simulink model "RBCM_Model"  (R2024b)
settings: Solver=FixedStepAuto  StartTime=0.0  StopTime=10.0  RelTol=1e-3
PreLoadFcn:
  | % NXP_MBDT_S32K3 callback: DO NOT REMOVE
  | mbd_s32k3.common.nxp.model_callbacks.preLoadFcn();
PostLoadFcn:
  | % NXP_MBDT_S32K3 callback: DO NOT REMOVE
  | mbd_s32k3.common.nxp.model_callbacks.postLoadFcn();
InitFcn:
  | % NXP_MBDT_S32K3 callback: DO NOT REMOVE
  | mbd_s32k3.common.nxp.model_callbacks.initFcn();
undefined symbols (not defined in the file or in its folder): AccuFanPwr_hHsd3ch2, BspdPwr_lHsd1ch2, BuzzerPwr_lHsd3ch3, DevicePwr_12v_lHsd1ch1, DevicePwr_hHsd1ch2, DrsPwr_8v_lHsd3ch1, hHsd_Diagnose_AdcBuffer, ILPwr_hHsd1ch1, lHsd_Diagnose_AdcBuffer, LoggerPwr_lHsd1ch3, PumpFan1_hHsd4ch1, PumpFan2_hHsd4ch2, PumpPwr_hHsd3ch1, RGBLED0state, TaillightPwr_lHsd3ch4, TempSensorPwr_lHsd1ch4
libraries: mbd_s32k3_io_library x127, simulink x48, canmsglib x8, mbd_s32k3_communication_library x7, mbd_s32k3_isr_library x6, mbd_s32k3_cdd_library x3, mbd_s32k3_utility_library x1
(part 8 of 10)

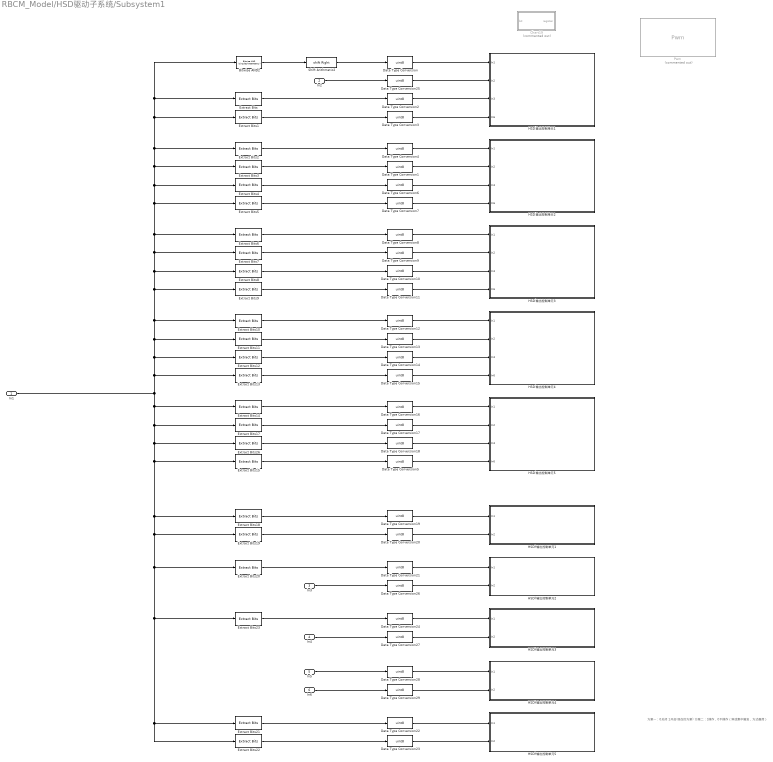
== system RBCM_Model/HSD驱动子系统/Subsystem1 ==
  note: 方案一：0关闭 1开启(现在的方案)
      | 方案二：1操作，0不操作（异或集中触发，方式最简）
  In1 : Inport  OutDataTypeStr=uint32
  In2 : Inport  Port=2  OutDataTypeStr=uint8
  In3 : Inport  Port=3  OutDataTypeStr=uint8
  In4 : Inport  Port=4  OutDataTypeStr=uint8
  In5 : Inport  Port=5  OutDataTypeStr=uint8
  In6 : Inport  Port=6  OutDataTypeStr=uint8
  Bitwise AND2 : simulink/Logic and Bit Operations/Bitwise Operator  logicop=AND  UseBitMask=on  BitMask=bin2dec('00000001')  BitMaskRealWorld=Stored Integer
      settings: LibrarySourceBlock=|
      | simulink/Quick Insert/Logic and Bit
      | Operations/Bitwise AND
  Chart19 : Stateflow chart  Commented=on  TreatAsAtomicUnit=on
  Data Type Conversion{,1..29} (30 alike) : DataTypeConversion  OutDataTypeStr=uint8  SaturateOnIntegerOverflow=off  RndMeth=Floor
  Extract Bits : simulink/Logic and Bit Operations/Extract Bits  bitsToExtract=Range of bits  numBits=8  bitIdxRange=[2 2]  outScalingMode=Preserve fixed-point scaling
  Extract Bits1 : simulink/Logic and Bit Operations/Extract Bits  bitsToExtract=Range of bits  numBits=8  bitIdxRange=[3 3]  outScalingMode=Preserve fixed-point scaling
  Extract Bits10 : simulink/Logic and Bit Operations/Extract Bits  bitsToExtract=Range of bits  numBits=8  bitIdxRange=[24 25]  outScalingMode=Preserve fixed-point scaling
  Extract Bits11 : simulink/Logic and Bit Operations/Extract Bits  bitsToExtract=Range of bits  numBits=8  bitIdxRange=[26 27]  outScalingMode=Preserve fixed-point scaling
  Extract Bits12 : simulink/Logic and Bit Operations/Extract Bits  bitsToExtract=Range of bits  numBits=8  bitIdxRange=[28 29]  outScalingMode=Preserve fixed-point scaling
  Extract Bits13 : simulink/Logic and Bit Operations/Extract Bits  bitsToExtract=Range of bits  numBits=8  bitIdxRange=[30 31]  outScalingMode=Preserve fixed-point scaling
  Extract Bits14 : simulink/Logic and Bit Operations/Extract Bits  bitsToExtract=Range of bits  numBits=8  bitIdxRange=[32 33]  outScalingMode=Preserve fixed-point scaling
  Extract Bits{15,18..23,26} (8 alike) : simulink/Logic and Bit Operations/Extract Bits  bitsToExtract=Range of bits  numBits=8  bitIdxRange=[36 37]  outScalingMode=Preserve fixed-point scaling
  Extract Bits17 : simulink/Logic and Bit Operations/Extract Bits  bitsToExtract=Range of bits  numBits=8  bitIdxRange=[34 35]  outScalingMode=Preserve fixed-point scaling
  Extract Bits2 : simulink/Logic and Bit Operations/Extract Bits  bitsToExtract=Range of bits  numBits=8  bitIdxRange=[4 4]  outScalingMode=Preserve fixed-point scaling
  Extract Bits3 : simulink/Logic and Bit Operations/Extract Bits  bitsToExtract=Range of bits  numBits=8  bitIdxRange=[5 5]  outScalingMode=Preserve fixed-point scaling
  Extract Bits4 : simulink/Logic and Bit Operations/Extract Bits  bitsToExtract=Range of bits  numBits=8  bitIdxRange=[6 6]  outScalingMode=Preserve fixed-point scaling
  Extract Bits5 : simulink/Logic and Bit Operations/Extract Bits  bitsToExtract=Range of bits  numBits=8  bitIdxRange=[7 7]  outScalingMode=Preserve fixed-point scaling
  Extract Bits6 : simulink/Logic and Bit Operations/Extract Bits  bitsToExtract=Range of bits  numBits=8  bitIdxRange=[16 17]  outScalingMode=Preserve fixed-point scaling
  Extract Bits7 : simulink/Logic and Bit Operations/Extract Bits  bitsToExtract=Range of bits  numBits=8  bitIdxRange=[18 19]  outScalingMode=Preserve fixed-point scaling
  Extract Bits8 : simulink/Logic and Bit Operations/Extract Bits  bitsToExtract=Range of bits  numBits=8  bitIdxRange=[20 21]  outScalingMode=Preserve fixed-point scaling
  Extract Bits9 : simulink/Logic and Bit Operations/Extract Bits  bitsToExtract=Range of bits  numBits=8  bitIdxRange=[22 23]  outScalingMode=Preserve fixed-point scaling
  HSDh输出控制单元1 : Subsystem
  HSDh输出控制单元2 : Subsystem
  HSDh输出控制单元3 : Subsystem
  HSDh输出控制单元4 : Subsystem
  HSDh输出控制单元5 : Subsystem
  HSDl输出控制单元1 : Subsystem
  HSDl输出控制单元2 : Subsystem
  HSDl输出控制单元3 : Subsystem
  HSDl输出控制单元4 : Subsystem
  HSDl输出控制单元5 : Subsystem
  Pwm : mbd_s32k3_io_library/Pwm  Commented=on  api_func=Pwm_SetDutyCycle  channel=PwmChannel_0  notification=PWM_RISING_EDGE  moduleId=PWM_EMIOS_INSTANCE_0  prescalerType=PWM_PRIMARY_PRESCALER  text=|
      | CommonPublishedInformation - CommonPublishedInformation Pwm 
      | CommonPublishedInformation/ArReleaseMajorVersion - 4 
      | CommonPublishedInformation/ArReleaseMinorVersion - 4 
      | CommonPublishedInformation/ArReleaseRevisionVersion - 0 
      | CommonPublishedInformation/ModuleId - 121 
      | CommonPublishedInformation/SwMajorVersion - 2 
      | CommonPublishedInformation/SwMinorVersion - 0 
      | CommonPublishedInformation/SwPatchVersion - 0 
      | CommonPublishedInformation/VendorId - 43 
      | IMPLEMENTATION-CONFIG-VARIANT - VARIANT-POST-BUILD 
      | POST_BUILD_VARIANT_USED - true 
      | PwmChannel - PwmChannel_0 PwmChannel_1 PwmChannel_2 PwmChannel_3 PwmChannel_4 PwmChannel_5 PwmChannel_6 PwmChannel_7 PwmChannel_8 
      | PwmChannel_0/Index - 0 
      | PwmChannel_0/PwmChannelId - 0 
      | PwmChannel_0/PwmDutycycleDefault - 2048 
      | PwmChannel_0/PwmHwChannel - /Pwm/Pwm/PwmChannelConfigSet/PwmEmios_0/PwmEmiosChannels_9 
      | PwmChannel_0/PwmIdleState - PWM_LOW 
      | PwmChannel_0/PwmMcuClockReferencePoint - /Mcu/Mcu/McuModuleConfiguration/McuClockSettingConfig_0/CORE_CLK 
      | PwmChannel_0/PwmNotification - PwmChannel_0_Callback 
      | PwmChannel_0/PwmPeriodDefault - 16000.0 
      | PwmChannel_0/PwmPeriodInTicks - true 
      | PwmChannel_0/PwmPolarity - PWM_HIGH 
      | PwmChannel_1/Index - 1 
      | PwmChannel_1/PwmChannelId - 1 
      | PwmChannel_1/PwmDutycycleDefault - 2048 
      | PwmChannel_1/PwmHwChannel - /Pwm/Pwm/PwmChannelConfigSet/PwmEmios_0/PwmEmiosChannels_17 
      | PwmChannel_1/PwmIdleState - PWM_LOW 
      | PwmChannel_1/PwmMcuClockReferencePoint - /Mcu/Mcu/McuModuleConfiguration/McuClockSettingConfig_0/CORE_CLK 
      | PwmChannel_1/PwmNotification - PwmChannel_1_Callback 
      | PwmChannel_1/PwmPeriodDefault - 16000.0 
      | PwmChannel_1/PwmPeriodInTicks - true 
      | PwmChannel_1/PwmPolarity - PWM_HIGH 
      | PwmChannel_2/Index - 2 
      | PwmChannel_2/PwmChannelId - 2 
      | PwmChannel_2/PwmDutycycleDefault - 0 
      | PwmChannel_2/PwmHwChannel - /Pwm/Pwm/PwmChannelConfigSet/PwmEmios_1/PwmEmiosChannels_19 
      | PwmChannel_2/PwmIdleState - PWM_LOW 
      | PwmChannel_2/PwmMcuClockReferencePoint - /Mcu/Mcu/McuModuleConfiguration/McuClockSettingConfig_0/CORE_CLK 
      | PwmChannel_2/PwmNotification - PwmChannel_2_Callback 
      | PwmChannel_2/PwmPeriodDefault - 16000.0 
      | PwmChannel_2/PwmPeriodInTicks - true 
      | PwmChannel_2/PwmPolarity - PWM_HIGH 
      | PwmChannel_3/Index - 3 
      | PwmChannel_3/PwmChannelId - 3 
      | PwmChannel_3/PwmDutycycleDefault - 0 
      | PwmChannel_3/PwmHwChannel - /Pwm/Pwm/PwmChannelConfigSet/PwmEmios_1/PwmEmiosChannels_20 
      | PwmChannel_3/PwmIdleState - PWM_LOW 
      | PwmChannel_3/PwmMcuClockReferencePoint - /Mcu/Mcu/McuModuleConfiguration/McuClockSettingConfig_0/CORE_CLK 
      | PwmChannel_3/PwmNotification - PwmChannel_3_Callback 
      | PwmChannel_3/PwmPeriodDefault - 16000.0 
      | PwmChannel_3/PwmPeriodInTicks - true 
      | PwmChannel_3/PwmPolarity - PWM_HIGH 
      | PwmChannel_4/Index - 4 
      | PwmChannel_4/PwmChannelId - 4 
      | PwmChannel_4/PwmDutycycleDefault - 0 
      | PwmChannel_4/PwmHwChannel - /Pwm/Pwm/PwmChannelConfigSet/PwmEmios_1/PwmEmiosChannels_0 
      | PwmChannel_4/PwmIdleState - PWM_LOW 
      | PwmChannel_4/PwmMcuClockReferencePoint - /Mcu/Mcu/McuModuleConfiguration/McuClockSettingConfig_0/CORE_CLK 
      | PwmChannel_4/PwmNotification - PwmChannel_4_Callback 
      | PwmChannel_4/PwmPeriodDefault - 16000.0 
      | PwmChannel_4/PwmPeriodInTicks - true 
      | PwmChannel_4/PwmPolarity - PWM_HIGH 
      | PwmChannel_5/Index - 5 
      | PwmChannel_5/PwmChannelId - 5 
      | PwmChannel_5/PwmDutycycleDefault - 0 
      | PwmChannel_5/PwmHwChannel - /Pwm/Pwm/PwmChannelConfigSet/PwmEmios_1/PwmEmiosChannels_1 
      | PwmChannel_5/PwmIdleState - PWM_LOW 
      | PwmChannel_5/PwmMcuClockReferencePoint - /Mcu/Mcu/McuModuleConfiguration/McuClockSettingConfig_0/CORE_CLK 
      | PwmChannel_5/PwmNotification - PwmChannel_5_Callback 
      | PwmChannel_5/PwmPeriodDefault - 16000.0 
      | PwmChannel_5/PwmPeriodInTicks - true 
      | PwmChannel_5/PwmPolarity - PWM_HIGH 
      | PwmChannel_6/Index - 6 
      | PwmChannel_6/PwmChannelId - 6 
      | PwmChannel_6/PwmDutycycleDefault - 0 
      | PwmChannel_6/PwmHwChannel - /Pwm/Pwm/PwmChannelConfigSet/PwmEmios_1/PwmEmiosChannels_21 
      | PwmChannel_6/PwmIdleState - PWM_LOW 
      | PwmChannel_6/PwmMcuClockReferencePoint - /Mcu/Mcu/McuModuleConfiguration/McuClockSettingConfig_0/CORE_CLK 
      | PwmChannel_6/PwmNotification - PwmChannel_6_Callback 
      | PwmChannel_6/PwmPeriodDefault - 16000.0 
      | PwmChannel_6/PwmPeriodInTicks - true 
      | PwmChannel_6/PwmPolarity - PWM_HIGH 
      | PwmChannel_7/Index - 7 
      | PwmChannel_7/PwmChannelId - 7 
      | PwmChannel_7/PwmDutycycleDefault - 0 
      | PwmChannel_7/PwmHwChannel - /Pwm/Pwm/PwmChannelConfigSet/PwmEmios_1/PwmEmiosChannels_22 
      | PwmChannel_7/PwmIdleState - PWM_LOW 
      | PwmChannel_7/PwmMcuClockReferencePoint - /Mcu/Mcu/McuModuleConfiguration/McuClockSettingConfig_0/CORE_CLK 
      | PwmChannel_7/PwmNotification - PwmChannel_7_Callback 
      | PwmChannel_7/PwmPeriodDefault - 16000.0 
      | PwmChannel_7/PwmPeriodInTicks - true 
      | PwmChannel_7/PwmPolarity - PWM_HIGH 
      | PwmChannel_8/Index - 8 
      | PwmChannel_8/PwmChannelId - 8 
      | PwmChannel_8/PwmDutycycleDefault - 0 
      | PwmChannel_8/PwmHwChannel - /Pwm/Pwm/PwmChannelConfigSet/PwmEmios_2/PwmEmiosChannels_7 
      | PwmChannel_8/PwmIdleState - PWM_LOW 
      | PwmChannel_8/PwmMcuClockReferencePoint - /Mcu/Mcu/McuModuleConfiguration/McuClockSettingConfig_0/CORE_CLK 
      | PwmChannel_8/PwmNotification - PwmChannel_8_Callback 
      | PwmChannel_8/PwmPeriodDefault - 40000 
      | PwmChannel_8/PwmPeriodInTicks - true 
      | PwmChannel_8/PwmPolarity - PWM_HIGH 
      | PwmConfigurationOfOptApiServices - PwmConfigurationOfOptApiServices 
      | PwmConfigurationOfOptApiServices/PwmDeInitApi - true 
      | PwmConfigurationOfOptApiServices/PwmEmiosFastUpdateApi - true 
      | PwmConfigurationOfOptApiServices/PwmEnableMaskOutputs - false 
      | PwmConfigurationOfOptApiServices/PwmGetChannelStateApi - true 
      | PwmConfigurationOfOptApiServices/PwmGetOutputState - true 
      | PwmConfigurationOfOptApiServices/PwmSetChannelDeadTime - true 
      | PwmConfigurationOfOptApiServices/PwmSetChannelOutputApi - true 
      | PwmConfigurationOfOptApiServices/PwmSetCounterBusApi - true 
      | PwmConfigurationOfOptApiServices/PwmSetDutyCycle - true 
      | PwmConfigurationOfOptApiServices/PwmSetDutyCycle_NoUpdate - false 
      | PwmConfigurationOfOptApiServices/PwmSetDutyPhaseShift - false 
      | PwmConfigurationOfOptApiServices/PwmSetOutputToIdle - true 
      | PwmConfigurationOfOptApiServices/PwmSetPeriodAndDuty - true 
      | PwmConfigurationOfOptApiServices/PwmSetPeriodAndDuty_NoUpdate - false 
      | PwmConfigurationOfOptApiServices/PwmSetTriggerDelayApi - true 
      | PwmConfigurationOfOptApiServices/PwmVersionInfoApi - true 
      | PwmEmios - PwmEmios_0 PwmEmios_1 PwmEmios_2 
      | PwmEmios_0/Index - 0 
      | PwmEmios_0/PwmEmiosChannels - PwmEmiosChannels_17 PwmEmiosChannels_9 
      | PwmEmios_0/PwmEmiosChannels_17/EmiosChCounterBus - EMIOS_PWM_IP_BUS_A 
      | PwmEmios_0/PwmEmiosChannels_17/EmiosChDeadtime - 0 
      | PwmEmios_0/PwmEmiosChannels_17/EmiosChFlagGeneration - Trailing_Edge 
      | PwmEmios_0/PwmEmiosChannels_17/EmiosChFreeze - false 
      | PwmEmios_0/PwmEmiosChannels_17/EmiosChId - CH_17 
      | PwmEmios_0/PwmEmiosChannels_17/EmiosChInterrupt - EMIOS_PWM_IP_INTERRUPT_REQUEST 
      | PwmEmios_0/PwmEmiosChannels_17/EmiosChMode - EMIOS_PWM_IP_MODE_OPWMB 
      | PwmEmios_0/PwmEmiosChannels_17/EmiosChOutputDisable - EMIOS_PWM_IP_OUTPUT_DISABLE_NONE 
      | PwmEmios_0/PwmEmiosChannels_17/EmiosChPhaseShift - 0 
      | PwmEmios_0/PwmEmiosChannels_17/EmiosChPrescaler - EMIOS_PWM_IP_CLOCK_DIV_2 
      | PwmEmios_0/PwmEmiosChannels_17/EmiosChPrescalerAlternate - EMIOS_PWM_IP_CLOCK_DIV_1 
      | PwmEmios_0/PwmEmiosChannels_17/EmiosChPrescalerSource - EMIOS_PWM_IP_PS_SRC_MODULE_CLOCK 
      | PwmEmios_0/PwmEmiosChannels_17/EmiosChTrigger - 0 
      | PwmEmios_0/PwmEmiosChannels_17/Index - 1 
      | PwmEmios_0/PwmEmiosChannels_17/PwmEmiosBusRef - /Mcl/Mcl/MclConfig/EmiosCommon_0/EmiosMclMasterBus_0 
      | PwmEmios_0/PwmEmiosChannels_9/EmiosChCounterBus - EMIOS_PWM_IP_BUS_A 
      | PwmEmios_0/PwmEmiosChannels_9/EmiosChDeadtime - 0 
      | PwmEmios_0/PwmEmiosChannels_9/EmiosChFlagGeneration - Trailing_Edge 
      | PwmEmios_0/PwmEmiosChannels_9/EmiosChFreeze - false 
      | PwmEmios_0/PwmEmiosChannels_9/EmiosChId - CH_9 
      | PwmEmios_0/PwmEmiosChannels_9/EmiosChInterrupt - EMIOS_PWM_IP_INTERRUPT_REQUEST 
      | PwmEmios_0/PwmEmiosChannels_9/EmiosChMode - EMIOS_PWM_IP_MODE_OPWMB 
      | PwmEmios_0/PwmEmiosChannels_9/EmiosChOutputDisable - EMIOS_PWM_IP_OUTPUT_DISABLE_NONE 
      | PwmEmios_0/PwmEmiosChannels_9/EmiosChPhaseShift - 0 
      | PwmEmios_0/PwmEmiosChannels_9/EmiosChPrescaler - EMIOS_PWM_IP_CLOCK_DIV_1 
      | PwmEmios_0/PwmEmiosChannels_9/EmiosChPrescalerAlternate - EMIOS_PWM_IP_CLOCK_DIV_1 
      | PwmEmios_0/PwmEmiosChannels_9/EmiosChPrescalerSource - EMIOS_PWM_IP_PS_SRC_MODULE_CLOCK 
      | PwmEmios_0/PwmEmiosChannels_9/EmiosChTrigger - 0 
      | PwmEmios_0/PwmEmiosChannels_9/Index - 0 
      | PwmEmios_0/PwmEmiosChannels_9/PwmEmiosBusRef - /Mcl/Mcl/MclConfig/EmiosCommon_0/EmiosMclMasterBus_0 
      | PwmEmios_0/PwmHwInstance - Emios_0 
      | PwmEmios_1/Index - 1 
      | PwmEmios_1/PwmEmiosChannels - PwmEmiosChannels_0 PwmEmiosChannels_1 PwmEmiosChannels_19 PwmEmiosChannels_20 PwmEmiosChannels_21 PwmEmiosChannels_22 
      | PwmEmios_1/PwmEmiosChannels_0/EmiosChCounterBus - EMIOS_PWM_IP_BUS_A 
      | PwmEmios_1/PwmEmiosChannels_0/EmiosChDeadtime - 0 
      | PwmEmios_1/PwmEmiosChannels_0/EmiosChFlagGeneration - Trailing_Edge 
      | PwmEmios_1/PwmEmiosChannels_0/EmiosChFreeze - false 
      | PwmEmios_1/PwmEmiosChannels_0/EmiosChId - CH_0 
      | PwmEmios_1/PwmEmiosChannels_0/EmiosChInterrupt - EMIOS_PWM_IP_INTERRUPT_REQUEST 
      | PwmEmios_1/PwmEmiosChannels_0/EmiosChMode - EMIOS_PWM_IP_MODE_OPWMB 
      | PwmEmios_1/PwmEmiosChannels_0/EmiosChOutputDisable - EMIOS_PWM_IP_OUTPUT_DISABLE_NONE 
      | PwmEmios_1/PwmEmiosChannels_0/EmiosChPhaseShift - 0 
      | PwmEmios_1/PwmEmiosChannels_0/EmiosChPrescaler - EMIOS_PWM_IP_CLOCK_DIV_1 
      | PwmEmios_1/PwmEmiosChannels_0/EmiosChPrescalerAlternate - EMIOS_PWM_IP_CLOCK_DIV_1 
      | PwmEmios_1/PwmEmiosChannels_0/EmiosChPrescalerSource - EMIOS_PWM_IP_PS_SRC_MODULE_CLOCK 
      | PwmEmios_1/PwmEmiosChannels_0/EmiosChTrigger - 0 
      | PwmEmios_1/PwmEmiosChannels_0/Index - 2 
      | PwmEmios_1/PwmEmiosChannels_0/PwmEmiosBusRef - /Mcl/Mcl/MclConfig/EmiosCommon_1/EmiosMclMasterBus_0 
      | PwmEmios_1/PwmEmiosChannels_1/EmiosChCounterBus - EMIOS_PWM_IP_BUS_A 
      | PwmEmios_1/PwmEmiosChannels_1/EmiosChDeadtime - 0 
      | PwmEmios_1/PwmEmiosChannels_1/EmiosChFlagGeneration - Trailing_Edge 
      | PwmEmios_1/PwmEmiosChannels_1/EmiosChFreeze - false 
      | PwmEmios_1/PwmEmiosChannels_1/EmiosChId - CH_1 
      | PwmEmios_1/PwmEmiosChannels_1/EmiosChInterrupt - EMIOS_PWM_IP_INTERRUPT_REQUEST 
      | PwmEmios_1/PwmEmiosChannels_1/EmiosChMode - EMIOS_PWM_IP_MODE_OPWMB 
      | PwmEmios_1/PwmEmiosChannels_1/EmiosChOutputDisable - EMIOS_PWM_IP_OUTPUT_DISABLE_NONE 
      | PwmEmios_1/PwmEmiosChannels_1/EmiosChPhaseShift - 0 
      | PwmEmios_1/PwmEmiosChannels_1/EmiosChPrescaler - EMIOS_PWM_IP_CLOCK_DIV_1 
      | PwmEmios_1/PwmEmiosChannels_1/EmiosChPrescalerAlternate - EMIOS_PWM_IP_CLOCK_DIV_1 
      | PwmEmios_1/PwmEmiosChannels_1/EmiosChPrescalerSource - EMIOS_PWM_IP_PS_SRC_MODULE_CLOCK 
      | PwmEmios_1/PwmEmiosChannels_1/EmiosChTrigger - 0 
      | PwmEmios_1/PwmEmiosChannels_1/Index - 3 
      | PwmEmios_1/PwmEmiosChannels_1/PwmEmiosBusRef - /Mcl/Mcl/MclConfig/EmiosCommon_1/EmiosMclMasterBus_0 
      | PwmEmios_1/PwmEmiosChannels_19/EmiosChCounterBus - EMIOS_PWM_IP_BUS_A 
      | PwmEmios_1/PwmEmiosChannels_19/EmiosChDeadtime - 0 
      | PwmEmios_1/PwmEmiosChannels_19/EmiosChFlagGeneration - Trailing_Edge 
      | PwmEmios_1/PwmEmiosChannels_19/EmiosChFreeze - false 
      | PwmEmios_1/PwmEmiosChannels_19/EmiosChId - CH_19 
      | PwmEmios_1/PwmEmiosChannels_19/EmiosChInterrupt - EMIOS_PWM_IP_INTERRUPT_REQUEST 
      | PwmEmios_1/PwmEmiosChannels_19/EmiosChMode - EMIOS_PWM_IP_MODE_OPWMB 
      | PwmEmios_1/PwmEmiosChannels_19/EmiosChOutputDisable - EMIOS_PWM_IP_OUTPUT_DISABLE_NONE 
      | PwmEmios_1/PwmEmiosChannels_19/EmiosChPhaseShift - 0 
      | PwmEmios_1/PwmEmiosChannels_19/EmiosChPrescaler - EMIOS_PWM_IP_CLOCK_DIV_1 
      | PwmEmios_1/PwmEmiosChannels_19/EmiosChPrescalerAlternate - EMIOS_PWM_IP_CLOCK_DIV_1 
      | PwmEmios_1/PwmEmiosChannels_19/EmiosChPrescalerSource - EMIOS_PWM_IP_PS_SRC_MODULE_CLOCK 
      | PwmEmios_1/PwmEmiosChannels_19/EmiosChTrigger - 0 
      | PwmEmios_1/PwmEmiosChannels_19/Index - 0 
      | PwmEmios_1/PwmEmiosChannels_19/PwmEmiosBusRef - /Mcl/Mcl/MclConfig/EmiosCommon_1/EmiosMclMasterBus_0 
      | PwmEmios_1/PwmEmiosChannels_20/EmiosChCounterBus - EMIOS_PWM_IP_BUS_A 
      | PwmEmios_1/PwmEmiosChannels_20/EmiosChDeadtime - 0 
      | PwmEmios_1/PwmEmiosChannels_20/EmiosChFlagGeneration - Trailing_Edge 
      | PwmEmios_1/PwmEmiosChannels_20/EmiosChFreeze - false 
      | PwmEmios_1/PwmEmiosChannels_20/EmiosChId - CH_20 
      | PwmEmios_1/PwmEmiosChannels_20/EmiosChInterrupt - EMIOS_PWM_IP_INTERRUPT_REQUEST 
      | PwmEmios_1/PwmEmiosChannels_20/EmiosChMode - EMIOS_PWM_IP_MODE_OPWMB 
      | PwmEmios_1/PwmEmiosChannels_20/EmiosChOutputDisable - EMIOS_PWM_IP_OUTPUT_DISABLE_NONE 
      | PwmEmios_1/PwmEmiosChannels_20/EmiosChPhaseShift - 0 
      | PwmEmios_1/PwmEmiosChannels_20/EmiosChPrescaler - EMIOS_PWM_IP_CLOCK_DIV_1 
      | PwmEmios_1/PwmEmiosChannels_20/EmiosChPrescalerAlternate - EMIOS_PWM_IP_CLOCK_DIV_1 
      | PwmEmios_1/PwmEmiosChannels_20/EmiosChPrescalerSource - EMIOS_PWM_IP_PS_SRC_MODULE_CLOCK 
      | PwmEmios_1/PwmEmiosChannels_20/EmiosChTrigger - 0 
      | PwmEmios_1/PwmEmiosChannels_20/Index - 1 
      | PwmEmios_1/PwmEmiosChannels_20/PwmEmiosBusRef - /Mcl/Mcl/MclConfig/EmiosCommon_1/EmiosMclMasterBus_0 
      | PwmEmios_1/PwmEmiosChannels_21/EmiosChCounterBus - EMIOS_PWM_IP_BUS_A 
      | PwmEmios_1/PwmEmiosChannels_21/EmiosChDeadtime - 0 
      | PwmEmios_1/PwmEmiosChannels_21/EmiosChFlagGeneration - Trailing_Edge 
      | PwmEmios_1/PwmEmiosChannels_21/EmiosChFreeze - false 
      | PwmEmios_1/PwmEmiosChannels_21/EmiosChId - CH_21 
      | PwmEmios_1/PwmEmiosChannels_21/EmiosChInterrupt - EMIOS_PWM_IP_INTERRUPT_REQUEST 
      | PwmEmios_1/PwmEmiosChannels_21/EmiosChMode - EMIOS_PWM_IP_MODE_OPWMB 
      | PwmEmios_1/PwmEmiosChannels_21/EmiosChOutputDisable - EMIOS_PWM_IP_OUTPUT_DISABLE_NONE 
      | PwmEmios_1/PwmEmiosChannels_21/EmiosChPhaseShift - 0 
      | PwmEmios_1/PwmEmiosChannels_21/EmiosChPrescaler - EMIOS_PWM_IP_CLOCK_DIV_1 
      | PwmEmios_1/PwmEmiosChannels_21/EmiosChPrescalerAlternate - EMIOS_PWM_IP_CLOCK_DIV_1 
      | PwmEmios_1/PwmEmiosChannels_21/EmiosChPrescalerSource - EMIOS_PWM_IP_PS_SRC_MODULE_CLOCK 
      | PwmEmios_1/PwmEmiosChannels_21/EmiosChTrigger - 0 
      | PwmEmios_1/PwmEmiosChannels_21/Index - 4 
      | PwmEmios_1/PwmEmiosChannels_21/PwmEmiosBusRef - /Mcl/Mcl/MclConfig/EmiosCommon_1/EmiosMclMasterBus_0 
      | PwmEmios_1/PwmEmiosChannels_22/EmiosChCounterBus - EMIOS_PWM_IP_BUS_A 
      | PwmEmios_1/PwmEmiosChannels_22/EmiosChDeadtime - 0 
      | PwmEmios_1/PwmEmiosChannels_22/EmiosChFlagGeneration - Trailing_Edge 
      | PwmEmios_1/PwmEmiosChannels_22/EmiosChFreeze - false 
      | PwmEmios_1/PwmEmiosChannels_22/EmiosChId - CH_22 
      | PwmEmios_1/PwmEmiosChannels_22/EmiosChInterrupt - EMIOS_PWM_IP_INTERRUPT_REQUEST 
      | PwmEmios_1/PwmEmiosChannels_22/EmiosChMode - EMIOS_PWM_IP_MODE_OPWMB 
      | PwmEmios_1/PwmEmiosChannels_22/EmiosChOutputDisable - EMIOS_PWM_IP_OUTPUT_DISABLE_NONE 
      | PwmEmios_1/PwmEmiosChannels_22/EmiosChPhaseShift - 0 
      | PwmEmios_1/PwmEmiosChannels_22/EmiosChPrescaler - EMIOS_PWM_IP_CLOCK_DIV_1 
      | PwmEmios_1/PwmEmiosChannels_22/EmiosChPrescalerAlternate - EMIOS_PWM_IP_CLOCK_DIV_1 
      | PwmEmios_1/PwmEmiosChannels_22/EmiosChPrescalerSource - EMIOS_PWM_IP_PS_SRC_MODULE_CLOCK 
      | PwmEmios_1/PwmEmiosChannels_22/EmiosChTrigger - 0 
      | PwmEmios_1/PwmEmiosChannels_22/Index - 5 
      | PwmEmios_1/PwmEmiosChannels_22/PwmEmiosBusRef - /Mcl/Mcl/MclConfig/EmiosCommon_1/EmiosMclMasterBus_0 
      | PwmEmios_1/PwmHwInstance - Emios_1 
      | PwmEmios_2/Index - 2 
      | PwmEmios_2/PwmEmiosChannels - PwmEmiosChannels_7 
      | PwmEmios_2/PwmEmiosChannels_7/EmiosChCounterBus - EMIOS_PWM_IP_BUS_A 
      | PwmEmios_2/PwmEmiosChannels_7/EmiosChDeadtime - 0 
      | PwmEmios_2/PwmEmiosChannels_7/EmiosChFlagGeneration - Trailing_Edge 
      | PwmEmios_2/PwmEmiosChannels_7/EmiosChFreeze - false 
      | PwmEmios_2/PwmEmiosChannels_7/EmiosChId - CH_7 
      | PwmEmios_2/PwmEmiosChannels_7/EmiosChInterrupt - EMIOS_PWM_IP_INTERRUPT_REQUEST 
      | PwmEmios_2/PwmEmiosChannels_7/EmiosChMode - EMIOS_PWM_IP_MODE_OPWMB 
      | PwmEmios_2/PwmEmiosChannels_7/EmiosChOutputDisable - EMIOS_PWM_IP_OUTPUT_DISABLE_NONE 
      | PwmEmios_2/PwmEmiosChannels_7/EmiosChPhaseShift - 0 
      | PwmEmios_2/PwmEmiosChannels_7/EmiosChPrescaler - EMIOS_PWM_IP_CLOCK_DIV_2 
      | PwmEmios_2/PwmEmiosChannels_7/EmiosChPrescalerAlternate - EMIOS_PWM_IP_CLOCK_DIV_2 
      | PwmEmios_2/PwmEmiosChannels_7/EmiosChPrescalerSource - EMIOS_PWM_IP_PS_SRC_MODULE_CLOCK 
      | PwmEmios_2/PwmEmiosChannels_7/EmiosChTrigger - 0 
      | PwmEmios_2/PwmEmiosChannels_7/Index - 0 
      | PwmEmios_2/PwmEmiosChannels_7/PwmEmiosBusRef - /Mcl/Mcl/MclConfig/EmiosCommon_2/EmiosMclMasterBus_0 
      | PwmEmios_2/PwmHwInstance - Emios_2 
      | PwmEtpu - PwmChannelConfigSet 
      | PwmGeneral - PwmGeneral 
      | PwmGeneral/PwmDevErrorDetect - true 
      | PwmGeneral/PwmDutycycleUpdatedEndperiod - false 
      | PwmGeneral/PwmEnableDualClockMode - false 
      | PwmGeneral/PwmEnableUserModeSupport - false 
      | PwmGeneral/PwmIndex - 0 
      | PwmGeneral/PwmMultiChannelSync - false 
      | PwmGeneral/PwmMultipartitionEnabled - false 
      | PwmGeneral/PwmNotificationSupported - true 
      | PwmGeneral/PwmPeriodUpdatedEndperiod - true
      settings: SourceProductName=IO Blocks
  Shift Arithmetic2 : ArithShift  BitShiftDirection=Right
  wires:
  Extract Bits22/1 -> Data Type Conversion23/1
  Data Type Conversion8/1 -> HSDl输出控制单元3/1(In1)
  Data Type Conversion23/1 -> HSDh输出控制单元5/2(In2)
  In5/1 -> Data Type Conversion28/1
  Data Type Conversion10/1 -> HSDl输出控制单元3/3(In3)
  Data Type Conversion3/1 -> HSDl输出控制单元1/4(In6)
  Data Type Conversion4/1 -> HSDl输出控制单元2/1(In1)
  Extract Bits8/1 -> Data Type Conversion10/1
  Extract Bits20/1 -> Data Type Conversion21/1
  Extract Bits2/1 -> Data Type Conversion4/1
  Data Type Conversion14/1 -> HSDl输出控制单元4/3(In3)
  Data Type Conversion6/1 -> HSDl输出控制单元2/3(In3)
  Extract Bits11/1 -> Data Type Conversion13/1
  Data Type Conversion15/1 -> HSDl输出控制单元4/4(In6)
  Extract Bits7/1 -> Data Type Conversion9/1
  Data Type Conversion27/1 -> HSDh输出控制单元3/2(In2)
  Extract Bits15/1 -> Data Type Conversion5/1
  Data Type Conversion22/1 -> HSDh输出控制单元5/1(In1)
  Data Type Conversion16/1 -> HSDl输出控制单元5/1(In1)
  Extract Bits5/1 -> Data Type Conversion7/1
  In2/1 -> Data Type Conversion25/1
  Data Type Conversion18/1 -> HSDl输出控制单元5/3(In3)
  Extract Bits26/1 -> Data Type Conversion18/1
  Extract Bits3/1 -> Data Type Conversion1/1
  In6/1 -> Data Type Conversion29/1
  Data Type Conversion/1 -> HSDl输出控制单元1/1(In1)
  Data Type Conversion24/1 -> HSDh输出控制单元3/1(In1)
  Data Type Conversion1/1 -> HSDl输出控制单元2/2(In2)
  Bitwise AND2/1 -> Shift Arithmetic2/1
  Extract Bits9/1 -> Data Type Conversion11/1
  Data Type Conversion9/1 -> HSDl输出控制单元3/2(In2)
  Extract Bits14/1 -> Data Type Conversion16/1
  Data Type Conversion21/1 -> HSDh输出控制单元2/1(In1)
  Data Type Conversion17/1 -> HSDl输出控制单元5/2(In2)
  Data Type Conversion19/1 -> HSDh输出控制单元1/1(In1)
  Data Type Conversion26/1 -> HSDh输出控制单元2/2(In2)
  Extract Bits21/1 -> Data Type Conversion22/1
  Shift Arithmetic2/1 -> Data Type Conversion/1
  Data Type Conversion5/1 -> HSDl输出控制单元5/4(In6)
  Extract Bits13/1 -> Data Type Conversion15/1
  Data Type Conversion7/1 -> HSDl输出控制单元2/4(In6)
  Extract Bits18/1 -> Data Type Conversion19/1
  Data Type Conversion11/1 -> HSDl输出控制单元3/4(In6)
  Extract Bits1/1 -> Data Type Conversion3/1
  Extract Bits4/1 -> Data Type Conversion6/1
  In1/1 -> Extract Bits26/1, Extract Bits15/1, Extract Bits18/1, Extract Bits22/1, Extract Bits21/1, Extract Bits23/1, Extract Bits20/1, Extract Bits19/1, Extract Bits17/1, Extract Bits14/1, Extract Bits13/1, Extract Bits12/1, Extract Bits11/1, Extract Bits10/1, Extract Bits9/1, Extract Bits8/1, Extract Bits7/1, Extract Bits6/1, Extract Bits5/1, Extract Bits4/1, Extract Bits3/1, Extract Bits2/1, Extract Bits/1, Bitwise AND2/1, Extract Bits1/1
  Extract Bits17/1 -> Data Type Conversion17/1
  Data Type Conversion2/1 -> HSDl输出控制单元1/3(In3)
  Data Type Conversion25/1 -> HSDl输出控制单元1/2(In2)
  Data Type Conversion29/1 -> HSDh输出控制单元4/2(In2)
  Extract Bits19/1 -> Data Type Conversion20/1
  Extract Bits/1 -> Data Type Conversion2/1
  Extract Bits6/1 -> Data Type Conversion8/1
  Data Type Conversion28/1 -> HSDh输出控制单元4/1(In1)
  Extract Bits12/1 -> Data Type Conversion14/1
  Data Type Conversion12/1 -> HSDl输出控制单元4/1(In1)
  In4/1 -> Data Type Conversion27/1
  Extract Bits23/1 -> Data Type Conversion24/1
  Extract Bits10/1 -> Data Type Conversion12/1
  In3/1 -> Data Type Conversion26/1
  Data Type Conversion13/1 -> HSDl输出控制单元4/2(In2)
  Data Type Conversion20/1 -> HSDh输出控制单元1/2(In2)

== system RBCM_Model/Subsystem13/Subsystem ==
  Action Port : ActionPort  ActionPortLabel=else
  HsdDriveCommand Struct1 : MATLAB Function  TreatAsAtomicUnit=on
  y : Outport
  wires:
  HsdDriveCommand Struct1/1(HsdDriveCommands) -> y/1

== system RBCM_Model/Subsystem13/Subsystem13 ==
  In1 : Inport
  Action Port : ActionPort  ActionPortLabel=if(u1 > 0)
  Out1 : Outport
  wires:
  In1/1 -> Out1/1

== system RBCM_Model/Subsystem5/Subsystem ==
  Action Port : ActionPort  ActionPortLabel=else
  MATLAB Function : MATLAB Function  TreatAsAtomicUnit=on
  y : Outport
  wires:
  MATLAB Function/1(y) -> y/1

== system RBCM_Model/Subsystem5/Subsystem13 ==
  In1 : Inport
  Action Port : ActionPort  ActionPortLabel=if(u1 > 0)
  Out1 : Outport
  wires:
  In1/1 -> Out1/1

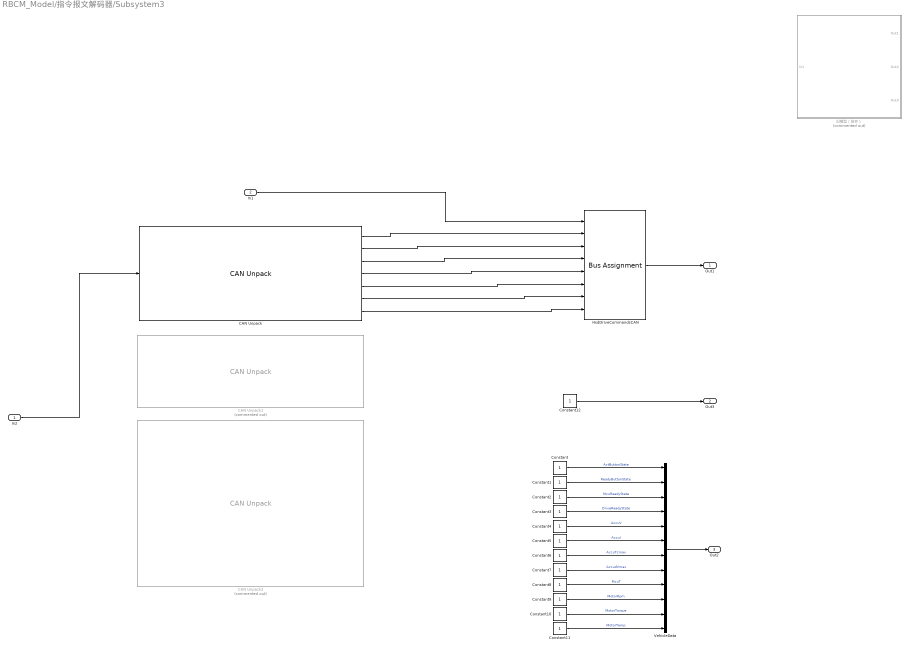
== system RBCM_Model/指令报文解码器/Subsystem3 ==
  In2 : Inport  OutDataTypeStr=Bus: Bus_CAN_RX_MESSAG
  In1 : Inport  Port=2
  CAN Unpack : canmsglib/CAN Unpack  CANdbFile=E:\Workspace\Myworkspace\RBCM_S32K344_AUTOSAR_MBD\Firmware\AUTOSAR_MBD\RBCM_ModelConfig\E10_dbc_240819_CAN.dbc  MsgList=PDB_ctr  MsgName=PDB_ctr  MsgIDType=Extended (29-bit identifier)  MsgIdentifier=514  MsgLength=8  SignalInfo={'Beep','2','2','LE','unsigned','Standard','0','1','0','0','2';'DRS','0','2','LE','unsigned','Standard','0','1','0','0','2';'FAN1','8','8','LE','unsigned','Standard','0','1','0','0','100';'FAN2','16','8','LE','unsigned','Standard','0','1','0','0','100';'FAN3','24','8','LE','unsigned','Standard','0','1','0','0','100';'Pump','40','8','LE','unsigned','Standard','0','1','0','0','100';'Taillight','32','8','LE','unsigned','Standard','0','1','0','0','100'}  IDPort=off  TimestampPort=off  ErrorPort=off  RemotePort=off  LengthPort=off  StatusPort=off  ApplyMinMax=off
      settings: LibrarySourceBlock=canlib/CAN Unpack  DataFormat=CANdb specified signals
  CAN Unpack1 : canmsglib/CAN Unpack  Commented=on  CANdbFile=E:\WUTE\整车CAN通信\E10_240721.dbc  MsgList=(none)  MsgName=MCU_Pwr  MsgIDType=Extended (29-bit identifier)  MsgIdentifier=218089455  MsgLength=8  SignalInfo={'MCU_HvAcCurrRms','48','16','LE','unsigned','Standard','0','0.1','-1600','-1600','1600';'MCU_HvCurr','32','16','LE','unsigned','Standard','0','0.1','-1600','-1600','1600';'MCU_HvVolt','16','16','LE','unsigned','Standard','0','0.1','0','0','1000';'MCU_McuTemp','0','8','LE','unsigned','Standard','0','1','-50','-50','205';'MCU_MotorTemp','8','8','LE','unsigned','Standard','0','1','-50','-50','205'}  IDPort=off  TimestampPort=off  ErrorPort=off  RemotePort=off  LengthPort=off  StatusPort=off  ApplyMinMax=off
      settings: LibrarySourceBlock=canlib/CAN Unpack  DataFormat=CANdb specified signals
  CAN Unpack2 : canmsglib/CAN Unpack  Commented=on  CANdbFile=E:\WUTE\整车CAN通信\E10_240721.dbc  MsgList=(none)  MsgName=MCU_Stat  MsgIDType=Extended (29-bit identifier)  MsgIdentifier=218089199  MsgLength=8  SignalInfo={'MCU_AlmLv','56','2','LE','unsigned','Standard','0','1','0','0','3';'MCU_IsBrakeMode','35','1','LE','unsigned','Standard','0','1','0','0','1';'MCU_IsFreeMode','32','1','LE','unsigned','Standard','0','1','0','0','1';'MCU_IsHvOvervoltage','44','1','LE','unsigned','Standard','0','1','0','0','1';'MCU_IsHvUndervoltage','46','1','LE','unsigned','Standard','0','1','0','0','1';'MCU_IsLvError','45','1','LE','unsigned','Standard','0','1','0','0','1';'MCU_IsMcuNOTActive','39','1','LE','unsigned','Standard','0','1','0','0','1';'MCU_IsMcuOvertemp','48','1','LE','unsigned','Standard','0','1','0','0','1';'MCU_IsMotorOvertemp','49','1','LE','unsigned','Standard','0','1','0','0','1';'MCU_IsOverCurr','43','1','LE','unsigned','Standard','0','1','0','0','1';'MCU_IsPreChg','41','1','LE','unsigned','Standard','0','1','0','0','255';'MCU_IsReady','40','1','LE','unsigned','Standard','0','1','0','0','1';'MCU_IsRevoloverError','42','1','LE','unsigned','Standard','0','1','0','0','1';'MCU_IsSelfcheckPass','55','1','LE','unsigned','Standard','0','1','0','0','1';'MCU_IsSpdMode','34','1','LE','unsigned','Standard','0','1','0','0','1';'MCU_IsTorqMode','33','1','LE','unsigned','Standard','0','1','0','0','1';'MCU_IsUnderPowerLim','47','1','LE','unsigned','Standard','0','1','0','0','1';'MCU_IsZeroLocMode','36','1','LE','unsigned','Standard','0','1','0','0','1';'MCU_SPD_RPT','0','16','LE','unsigned','Standard','0','0.5','-10000','-10000','10000';'MCU_TORQ_RPT','16','16','LE','unsigned','Standard','0','1','0','0','1000'}  IDPort=off  TimestampPort=off  ErrorPort=off  RemotePort=off  LengthPort=off  StatusPort=off  ApplyMinMax=off
      settings: LibrarySourceBlock=canlib/CAN Unpack  DataFormat=CANdb specified signals
  Constant{,1..3,12} (5 alike) : Constant  OutDataTypeStr=uint8
  Constant{4..11} (8 alike) : Constant  OutDataTypeStr=uint16
  HsdDriveCommandsCAN : BusAssignment  AssignedSignals=BuzzerPwr_lHsd3ch3,DrsPwr_8v_lHsd3ch1,AccuFanPwr_hHsd3ch2,PumpFan1_hHsd4ch1,PumpFan2_hHsd4ch2,PumpPwr_hHsd3ch1,TaillightPwr_lHsd3ch4
  VehicleData : BusCreator  Inputs=12  OutDataTypeStr=Bus: Bus_Vehicle_Data  NonVirtualBus=on
      settings: InheritFromInputs=off
  旧模型（放弃） : Subsystem  Commented=on
  Out1 : Outport
  Out3 : Outport  Port=2
  Out2 : Outport  Port=3
  wires:
  In2/1 -> CAN Unpack/1
  In1/1 -> HsdDriveCommandsCAN/1
  CAN Unpack/1 -> HsdDriveCommandsCAN/2
  CAN Unpack/2 -> HsdDriveCommandsCAN/3
  CAN Unpack/3 -> HsdDriveCommandsCAN/4
  CAN Unpack/4 -> HsdDriveCommandsCAN/5
  CAN Unpack/5 -> HsdDriveCommandsCAN/6
  CAN Unpack/6 -> HsdDriveCommandsCAN/7
  CAN Unpack/7 -> HsdDriveCommandsCAN/8
  HsdDriveCommandsCAN/1 -> Out1/1
  VehicleData/1 -> Out2/1
  Constant/1 -> VehicleData/1  "ActButtonState"
  Constant1/1 -> VehicleData/2  "ReadyButtonState"
  Constant2/1 -> VehicleData/3  "McuReadyState"
  Constant3/1 -> VehicleData/4  "DriveReadyState"
  Constant4/1 -> VehicleData/5  "AccuV"
  Constant5/1 -> VehicleData/6  "AccuI"
  Constant6/1 -> VehicleData/7  "AccuTcmax"
  Constant7/1 -> VehicleData/8  "AccudVmax"
  Constant8/1 -> VehicleData/9  "McuT"
  Constant9/1 -> VehicleData/10  "MotorRpm"
  Constant10/1 -> VehicleData/11  "MotorTorque"
  Constant11/1 -> VehicleData/12  "MotorTemp"
  Constant12/1 -> Out3/1

== system RBCM_Model/无线调试模式管理子系统/Subsystem ==
  Action Port : ActionPort  ActionPortLabel=if(u1 == 0)
  Constant : Constant  OutDataTypeStr=uint8
  Constant1 : Constant  OutDataTypeStr=uint8
  Dio : mbd_s32k3_io_library/Dio  api_func=Dio_WriteChannel  channel=ESP32S3_EN_RESET  channel_group=No channel groups configured  port=PTB_H  gpioSim=on  text=<binary blob, 15399 chars, not shown>
      settings: SourceProductName=IO Blocks
  Dio1 : mbd_s32k3_io_library/Dio  api_func=Dio_WriteChannel  channel=ESP32S3_EN_SET  channel_group=No channel groups configured  port=PTB_H  gpioSim=on  text=<binary blob, 15399 chars, not shown>
      settings: SourceProductName=IO Blocks
  wires:
  Constant/1 -> Dio/1
  Constant1/1 -> Dio1/1

== system RBCM_Model/无线调试模式管理子系统/Subsystem1 ==
  Action Port : ActionPort  ActionPortLabel=else
  Constant : Constant  Value=0  OutDataTypeStr=uint8
  Dio : mbd_s32k3_io_library/Dio  api_func=Dio_WriteChannel  channel=ESP32S3_EN_RESET  channel_group=No channel groups configured  port=PTB_H  gpioSim=on  text=<binary blob, 15399 chars, not shown>
      settings: SourceProductName=IO Blocks
  wires:
  Constant/1 -> Dio/1

== system RBCM_Model/HSD诊断分析子系统/旧模型/ADC采集与处理单元11 ==
  note: 计算设备工作电流
  note: 计算ADC输入实际电压
  note: 计算设备功耗
  function : TriggerPort  TriggerType=function-call  VariantControl=Variant
  ADC resolution : Constant  Value=0b111111111111  OutDataTypeStr=uint16
  Data Store Read : DataStoreRead  DataStoreName=hHsd_Diagnose_AdcBuffer  DataStoreElements=hHsd_Diagnose_AdcBuffer(1)  IndexOptions=Index vector (dialog)  Indices=1  OutputSizes=1
  Data Type Conversion : DataTypeConversion  OutDataTypeStr=single  SaturateOnIntegerOverflow=off  RndMeth=Floor
  Divide : Product  Inputs=*/  OutDataTypeStr=single
  Magnification : Gain  Gain=1450  OutDataTypeStr=uint8
  Product : Product  OutDataTypeStr=single
  Product1 : Product  OutDataTypeStr=single
  Product2 : Product  OutDataTypeStr=single
  Ris : Constant  Value=650  OutDataTypeStr=uint16
  Subtract : Sum  Inputs=+-
  Terminator7 : Terminator
  Vbat : Constant  Value=28  OutDataTypeStr=uint16
  Vref : Constant  Value=5  OutDataTypeStr=uint8
  compensate : Constant  Value=0.05  OutDataTypeStr=single
  u : Outport
  wires:
  Data Store Read/1 -> Data Type Conversion/1
  Data Type Conversion/1 -> Product/1
  Product2/1 -> Terminator7/1  "device power value"
  compensate/1 -> Subtract/2
  Product1/1 -> Divide/1  "Actual voltage"
  Vbat/1 -> Subtract/1
  Product/1 -> Product1/2
  Vref/1 -> Product1/1
  Subtract/1 -> Product2/2
  Divide/1 -> Magnification/1
  Ris/1 -> Divide/2
  ADC resolution/1 -> Product/2
  Magnification/1 -> u/1, Product2/1  "device current value"

== system RBCM_Model/HSD诊断分析子系统/旧模型/ADC采集与处理单元2 ==
  note: 计算ADC输入实际电压
  note: 计算设备工作电流*10
  note: 计算设备功耗
  function : TriggerPort  TriggerType=function-call  VariantControl=Variant
  ADC resolution : Constant  Value=0b111111111111  OutDataTypeStr=uint16
  Data Store Read : DataStoreRead  DataStoreName=lHsd_Diagnose_AdcBuffer  DataStoreElements=lHsd_Diagnose_AdcBuffer(2)  IndexOptions=Index vector (dialog)  Indices=1  OutputSizes=1
  Data Type Conversion : DataTypeConversion  OutDataTypeStr=single  SaturateOnIntegerOverflow=off  RndMeth=Floor
  Divide : Product  Inputs=*/  OutDataTypeStr=single
  Magnification : Gain  Gain=300  OutDataTypeStr=uint8
  Product : Product  OutDataTypeStr=single
  Product1 : Product  OutDataTypeStr=single
  Product2 : Product  OutDataTypeStr=single
  Ris : Constant  Value=650  OutDataTypeStr=uint16
  Subtract : Sum  Inputs=+-
  Terminator7 : Terminator
  Vbat : Constant  Value=28  OutDataTypeStr=uint16
  Vref : Constant  Value=5  OutDataTypeStr=uint8
  compensate : Constant  Value=0.05  OutDataTypeStr=single
  u1 : Outport  OutDataTypeStr=uint8
  wires:
  Data Type Conversion/1 -> Product/1
  Product2/1 -> Terminator7/1  "device power value"
  Subtract/1 -> Product2/2
  compensate/1 -> Subtract/2
  Vbat/1 -> Subtract/1
  ADC resolution/1 -> Product/2
  Product/1 -> Product1/2
  Vref/1 -> Product1/1
  Product1/1 -> Divide/1  "Actual voltage"
  Ris/1 -> Divide/2
  Divide/1 -> Magnification/1
  Magnification/1 -> Product2/1, u1/1  "device current value"
  Data Store Read/1 -> Data Type Conversion/1

== system RBCM_Model/HSD诊断分析子系统/旧模型/ADC采集与处理单元3 ==
  note: 计算设备功耗
  note: 计算设备工作电流*10
  note: 计算ADC输入实际电压
  function : TriggerPort  TriggerType=function-call  VariantControl=Variant
  ADC resolution : Constant  Value=0b111111111111  OutDataTypeStr=uint16
  Data Store Read : DataStoreRead  DataStoreName=lHsd_Diagnose_AdcBuffer  DataStoreElements=lHsd_Diagnose_AdcBuffer(3)  IndexOptions=Index vector (dialog)  Indices=1  OutputSizes=1
  Data Type Conversion : DataTypeConversion  OutDataTypeStr=single  SaturateOnIntegerOverflow=off  RndMeth=Floor
  Divide : Product  Inputs=*/  OutDataTypeStr=single
  Magnification : Gain  Gain=300  OutDataTypeStr=uint8
  Product : Product  OutDataTypeStr=single
  Product1 : Product  OutDataTypeStr=single
  Product2 : Product  OutDataTypeStr=single
  Ris : Constant  Value=650  OutDataTypeStr=uint16
  Subtract : Sum  Inputs=+-
  Terminator7 : Terminator
  Vbat : Constant  Value=28  OutDataTypeStr=uint16
  Vref : Constant  Value=5  OutDataTypeStr=uint8
  compensate : Constant  Value=0.05  OutDataTypeStr=single
  u1 : Outport  OutDataTypeStr=uint8
  wires:
  Magnification/1 -> u1/1, Product2/1  "device current value"
  Divide/1 -> Magnification/1
  Ris/1 -> Divide/2
  Product1/1 -> Divide/1  "Actual voltage"
  Vref/1 -> Product1/1
  Product/1 -> Product1/2
  ADC resolution/1 -> Product/2
  Data Store Read/1 -> Data Type Conversion/1
  Vbat/1 -> Subtract/1
  compensate/1 -> Subtract/2
  Subtract/1 -> Product2/2
  Product2/1 -> Terminator7/1  "device power value"
  Data Type Conversion/1 -> Product/1

== system RBCM_Model/HSD诊断分析子系统/旧模型/ADC采集与处理单元4 ==
  note: 计算ADC输入实际电压
  note: 计算设备工作电流*10
  note: 计算设备功耗
  function : TriggerPort  TriggerType=function-call  VariantControl=Variant
  ADC resolution : Constant  Value=0b111111111111  OutDataTypeStr=uint16
  Data Store Read : DataStoreRead  DataStoreName=lHsd_Diagnose_AdcBuffer  DataStoreElements=lHsd_Diagnose_AdcBuffer(4)  IndexOptions=Index vector (dialog)  Indices=1  OutputSizes=1
  Data Type Conversion : DataTypeConversion  OutDataTypeStr=single  SaturateOnIntegerOverflow=off  RndMeth=Floor
  Divide : Product  Inputs=*/  OutDataTypeStr=single
  Magnification : Gain  Gain=300  OutDataTypeStr=uint8
  Product : Product  OutDataTypeStr=single
  Product1 : Product  OutDataTypeStr=single
  Product2 : Product  OutDataTypeStr=single
  Ris : Constant  Value=650  OutDataTypeStr=uint16
  Subtract : Sum  Inputs=+-
  Terminator7 : Terminator
  Vbat : Constant  Value=28  OutDataTypeStr=uint16
  Vref : Constant  Value=5  OutDataTypeStr=uint8
  compensate : Constant  Value=0.05  OutDataTypeStr=single
  u1 : Outport  OutDataTypeStr=uint8
  wires:
  Data Type Conversion/1 -> Product/1
  Product2/1 -> Terminator7/1  "device power value"
  Subtract/1 -> Product2/2
  compensate/1 -> Subtract/2
  Vbat/1 -> Subtract/1
  Data Store Read/1 -> Data Type Conversion/1
  ADC resolution/1 -> Product/2
  Product/1 -> Product1/2
  Vref/1 -> Product1/1
  Product1/1 -> Divide/1  "Actual voltage"
  Ris/1 -> Divide/2
  Divide/1 -> Magnification/1
  Magnification/1 -> Product2/1, u1/1  "device current value"

== system RBCM_Model/HSD诊断分析子系统/旧模型/ADC采集与处理单元5 ==
  note: 计算设备功耗
  note: 计算设备工作电流*10
  note: 计算ADC输入实际电压
  function : TriggerPort  TriggerType=function-call  VariantControl=Variant
  ADC resolution : Constant  Value=0b111111111111  OutDataTypeStr=uint16
  Data Store Read : DataStoreRead  DataStoreName=lHsd_Diagnose_AdcBuffer  DataStoreElements=lHsd_Diagnose_AdcBuffer(5)  IndexOptions=Index vector (dialog)  Indices=1  OutputSizes=1
  Data Type Conversion : DataTypeConversion  OutDataTypeStr=single  SaturateOnIntegerOverflow=off  RndMeth=Floor
  Divide : Product  Inputs=*/  OutDataTypeStr=single
  Magnification : Gain  Gain=300  OutDataTypeStr=uint8
  Product : Product  OutDataTypeStr=single
  Product1 : Product  OutDataTypeStr=single
  Product2 : Product  OutDataTypeStr=single
  Ris : Constant  Value=650  OutDataTypeStr=uint16
  Subtract : Sum  Inputs=+-
  Terminator7 : Terminator
  Vbat : Constant  Value=28  OutDataTypeStr=uint16
  Vref : Constant  Value=5  OutDataTypeStr=uint8
  compensate : Constant  Value=0.05  OutDataTypeStr=single
  u1 : Outport  OutDataTypeStr=uint8
  wires:
  Magnification/1 -> u1/1, Product2/1  "device current value"
  Divide/1 -> Magnification/1
  Ris/1 -> Divide/2
  Product1/1 -> Divide/1  "Actual voltage"
  Vref/1 -> Product1/1
  Product/1 -> Product1/2
  ADC resolution/1 -> Product/2
  Data Store Read/1 -> Data Type Conversion/1
  Vbat/1 -> Subtract/1
  compensate/1 -> Subtract/2
  Subtract/1 -> Product2/2
  Product2/1 -> Terminator7/1  "device power value"
  Data Type Conversion/1 -> Product/1

== system RBCM_Model/HSD诊断分析子系统/旧模型/ADC采集与处理单元6 ==
  note: 计算设备功耗
  note: 计算ADC输入实际电压
  note: 计算设备工作电流
  function : TriggerPort  TriggerType=function-call  VariantControl=Variant
  ADC resolution : Constant  Value=0b111111111111  OutDataTypeStr=uint16
  Data Store Read : DataStoreRead  DataStoreName=hHsd_Diagnose_AdcBuffer  DataStoreElements=hHsd_Diagnose_AdcBuffer(2)  IndexOptions=Index vector (dialog)  Indices=1  OutputSizes=1
  Data Type Conversion : DataTypeConversion  OutDataTypeStr=single  SaturateOnIntegerOverflow=off  RndMeth=Floor
  Divide : Product  Inputs=*/  OutDataTypeStr=single
  Magnification : Gain  Gain=1450  OutDataTypeStr=uint8
  Product : Product  OutDataTypeStr=single
  Product1 : Product  OutDataTypeStr=single
  Product2 : Product  OutDataTypeStr=single
  Ris : Constant  Value=650  OutDataTypeStr=uint16
  Subtract : Sum  Inputs=+-
  Terminator7 : Terminator
  Vbat : Constant  Value=28  OutDataTypeStr=uint16
  Vref : Constant  Value=5  OutDataTypeStr=uint8
  compensate : Constant  Value=0.05  OutDataTypeStr=single
  u : Outport
  wires:
  Magnification/1 -> Product2/1, u/1  "device current value"
  ADC resolution/1 -> Product/2
  Ris/1 -> Divide/2
  Divide/1 -> Magnification/1
  Subtract/1 -> Product2/2
  Vref/1 -> Product1/1
  Product/1 -> Product1/2
  Vbat/1 -> Subtract/1
  Product1/1 -> Divide/1  "Actual voltage"
  compensate/1 -> Subtract/2
  Product2/1 -> Terminator7/1  "device power value"
  Data Type Conversion/1 -> Product/1
  Data Store Read/1 -> Data Type Conversion/1

== system RBCM_Model/HSD诊断分析子系统/旧模型/ADC采集与处理单元7 ==
  note: 计算设备工作电流
  note: 计算ADC输入实际电压
  note: 计算设备功耗
  function : TriggerPort  TriggerType=function-call  VariantControl=Variant
  ADC resolution : Constant  Value=0b111111111111  OutDataTypeStr=uint16
  Data Store Read : DataStoreRead  DataStoreName=hHsd_Diagnose_AdcBuffer  DataStoreElements=hHsd_Diagnose_AdcBuffer(3)  IndexOptions=Index vector (dialog)  Indices=1  OutputSizes=1
  Data Type Conversion : DataTypeConversion  OutDataTypeStr=single  SaturateOnIntegerOverflow=off  RndMeth=Floor
  Divide : Product  Inputs=*/  OutDataTypeStr=single
  Magnification : Gain  Gain=1450  OutDataTypeStr=uint8
  Product : Product  OutDataTypeStr=single
  Product1 : Product  OutDataTypeStr=single
  Product2 : Product  OutDataTypeStr=single
  Ris : Constant  Value=650  OutDataTypeStr=uint16
  Subtract : Sum  Inputs=+-
  Terminator7 : Terminator
  Vbat : Constant  Value=28  OutDataTypeStr=uint16
  Vref : Constant  Value=5  OutDataTypeStr=uint8
  compensate : Constant  Value=0.05  OutDataTypeStr=single
  u : Outport
  wires:
  Data Store Read/1 -> Data Type Conversion/1
  Data Type Conversion/1 -> Product/1
  Product2/1 -> Terminator7/1  "device power value"
  compensate/1 -> Subtract/2
  Product1/1 -> Divide/1  "Actual voltage"
  Vbat/1 -> Subtract/1
  Product/1 -> Product1/2
  Vref/1 -> Product1/1
  Subtract/1 -> Product2/2
  Divide/1 -> Magnification/1
  Ris/1 -> Divide/2
  ADC resolution/1 -> Product/2
  Magnification/1 -> u/1, Product2/1  "device current value"

== system RBCM_Model/HSD诊断分析子系统/旧模型/ADC采集与处理单元8 ==
  note: 计算设备功耗
  note: 计算ADC输入实际电压
  note: 计算设备工作电流
  function : TriggerPort  TriggerType=function-call  VariantControl=Variant
  ADC resolution : Constant  Value=0b111111111111  OutDataTypeStr=uint16
  Data Store Read : DataStoreRead  DataStoreName=hHsd_Diagnose_AdcBuffer  DataStoreElements=hHsd_Diagnose_AdcBuffer(4)  IndexOptions=Index vector (dialog)  Indices=1  OutputSizes=1
  Data Type Conversion : DataTypeConversion  OutDataTypeStr=single  SaturateOnIntegerOverflow=off  RndMeth=Floor
  Divide : Product  Inputs=*/  OutDataTypeStr=single
  Magnification : Gain  Gain=1450  OutDataTypeStr=uint8
  Product : Product  OutDataTypeStr=single
  Product1 : Product  OutDataTypeStr=single
  Product2 : Product  OutDataTypeStr=single
  Ris : Constant  Value=650  OutDataTypeStr=uint16
  Subtract : Sum  Inputs=+-
  Terminator7 : Terminator
  Vbat : Constant  Value=28  OutDataTypeStr=uint16
  Vref : Constant  Value=5  OutDataTypeStr=uint8
  compensate : Constant  Value=0.05  OutDataTypeStr=single
  u : Outport
  wires:
  Magnification/1 -> Product2/1, u/1  "device current value"
  ADC resolution/1 -> Product/2
  Ris/1 -> Divide/2
  Divide/1 -> Magnification/1
  Subtract/1 -> Product2/2
  Vref/1 -> Product1/1
  Product/1 -> Product1/2
  Vbat/1 -> Subtract/1
  Product1/1 -> Divide/1  "Actual voltage"
  compensate/1 -> Subtract/2
  Product2/1 -> Terminator7/1  "device power value"
  Data Type Conversion/1 -> Product/1
  Data Store Read/1 -> Data Type Conversion/1

== system RBCM_Model/HSD诊断分析子系统/旧模型/ADC采集与处理单元9 ==
  note: 计算设备工作电流
  note: 计算ADC输入实际电压
  note: 计算设备功耗
  function : TriggerPort  TriggerType=function-call  VariantControl=Variant
  ADC resolution : Constant  Value=0b111111111111  OutDataTypeStr=uint16
  Data Store Read : DataStoreRead  DataStoreName=hHsd_Diagnose_AdcBuffer  DataStoreElements=hHsd_Diagnose_AdcBuffer(5)  IndexOptions=Index vector (dialog)  Indices=1  OutputSizes=1
  Data Type Conversion : DataTypeConversion  OutDataTypeStr=single  SaturateOnIntegerOverflow=off  RndMeth=Floor
  Divide : Product  Inputs=*/  OutDataTypeStr=single
  Magnification : Gain  Gain=1450  OutDataTypeStr=uint8
  Product : Product  OutDataTypeStr=single
  Product1 : Product  OutDataTypeStr=single
  Product2 : Product  OutDataTypeStr=single
  Ris : Constant  Value=650  OutDataTypeStr=uint16
  Subtract : Sum  Inputs=+-
  Terminator7 : Terminator
  Vbat : Constant  Value=28  OutDataTypeStr=uint16
  Vref : Constant  Value=5  OutDataTypeStr=uint8
  compensate : Constant  Value=0.05  OutDataTypeStr=single
  u : Outport
  wires:
  Data Store Read/1 -> Data Type Conversion/1
  Data Type Conversion/1 -> Product/1
  Product2/1 -> Terminator7/1  "device power value"
  compensate/1 -> Subtract/2
  Product1/1 -> Divide/1  "Actual voltage"
  Vbat/1 -> Subtract/1
  Product/1 -> Product1/2
  Vref/1 -> Product1/1
  Subtract/1 -> Product2/2
  Divide/1 -> Magnification/1
  Ris/1 -> Divide/2
  ADC resolution/1 -> Product/2
  Magnification/1 -> u/1, Product2/1  "device current value"

== system RBCM_Model/HSD诊断分析子系统/旧模型/HSDh片选执行单元1 ==
  y : Inport
  Data Type Conversion4 : DataTypeConversion  OutDataTypeStr=boolean  SaturateOnIntegerOverflow=off  RndMeth=Floor
  Dio : mbd_s32k3_io_library/Dio  api_func=Dio_WriteChannel  channel=RGBLED0_BLUE  channel_group=No channel groups configured  port=PTB_H  gpioSim=on  text=<binary blob, 15399 chars, not shown>
      settings: SourceProductName=IO Blocks
  wires:
  Data Type Conversion4/1 -> Dio/1
  y/1 -> Data Type Conversion4/1

== system RBCM_Model/HSD诊断分析子系统/旧模型/HSDh片选执行单元11 ==
  y : Inport
  Data Type Conversion4 : DataTypeConversion  OutDataTypeStr=boolean  SaturateOnIntegerOverflow=off  RndMeth=Floor
  Dio : mbd_s32k3_io_library/Dio  api_func=Dio_WriteChannel  channel=RGBLED0_BLUE  channel_group=No channel groups configured  port=PTB_H  gpioSim=on  text=<binary blob, 15399 chars, not shown>
      settings: SourceProductName=IO Blocks
  wires:
  y/1 -> Data Type Conversion4/1
  Data Type Conversion4/1 -> Dio/1

== system RBCM_Model/HSD诊断分析子系统/旧模型/HSDh片选执行单元2 ==
  y : Inport
  Data Type Conversion4 : DataTypeConversion  OutDataTypeStr=boolean  SaturateOnIntegerOverflow=off  RndMeth=Floor
  Dio : mbd_s32k3_io_library/Dio  api_func=Dio_WriteChannel  channel=RGBLED0_BLUE  channel_group=No channel groups configured  port=PTB_H  gpioSim=on  text=<binary blob, 15399 chars, not shown>
      settings: SourceProductName=IO Blocks
  wires:
  y/1 -> Data Type Conversion4/1
  Data Type Conversion4/1 -> Dio/1
